simulink model "step05_STM32_ControllerPrep"  (R2024b)
settings: Solver=VariableStepAuto  StartTime=0.0  StopTime=1.5  RelTol=1e-3
libraries: spsSeriesRLCBranchLib x6, spsCurrentMeasurementLib x4, spsUniversalBridgeLib x2, spsVoltageMeasurementLib x2, spsACVoltageSourceLib x1, spsRMSLib x1, slpidlib x1, spspowerguiLib x1
settings Model: Creator=asus  LastModifiedBy=asus

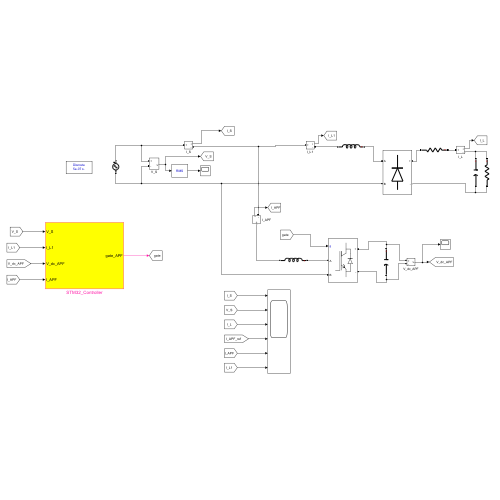
[thumbnail: Simulink's stored preview of the top-level diagram]
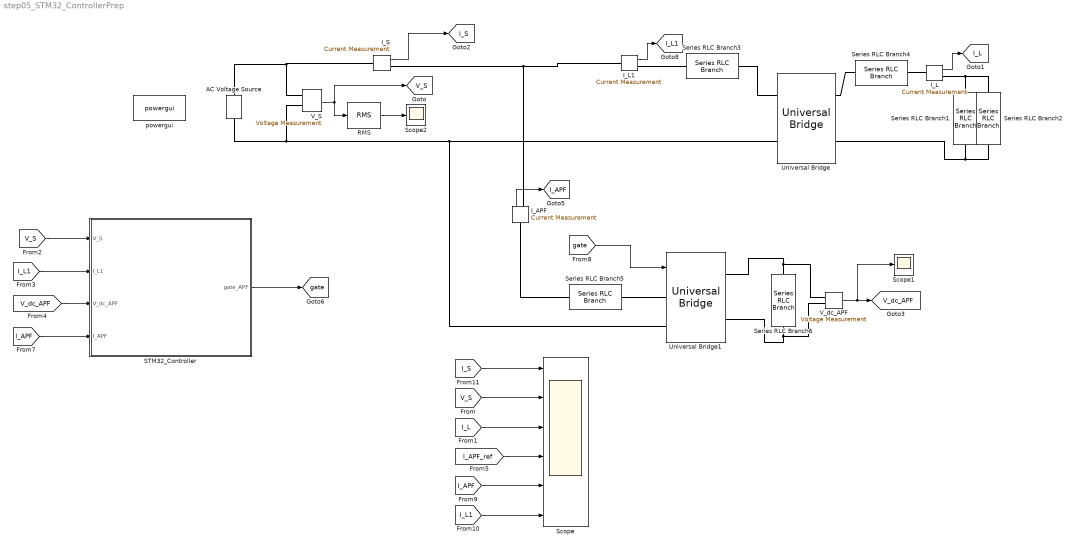
== system step05_STM32_ControllerPrep ==
  AC Voltage Source : spsACVoltageSourceLib/AC Voltage Source  Amplitude=67.88225  Phase=0  Frequency=50  SampleTime=0  Measurements=None  BusType=swing  Pref=10e3  Qref=0  Qmin=-inf  Qmax=+inf
  I_APF : spsCurrentMeasurementLib/Current Measurement  PhasorSimulation=off  OutputType=Complex  PSBequivalent=0
  I_L : spsCurrentMeasurementLib/Current Measurement  PhasorSimulation=off  OutputType=Complex  PSBequivalent=0
  I_L1 : spsCurrentMeasurementLib/Current Measurement  PhasorSimulation=off  OutputType=Complex  PSBequivalent=0
  I_S : spsCurrentMeasurementLib/Current Measurement  PhasorSimulation=off  OutputType=Complex  PSBequivalent=0
  RMS : spsRMSLib/RMS  TrueRMS=on  Freq=50  RMSInit=120  Ts=0
  STM32_Controller : Subsystem
  Scope : Scope  NumInputPorts=6
  Scope1 : Scope
  Scope2 : Scope
  Series RLC Branch1 : spsSeriesRLCBranchLib/Series RLC Branch  LConnTagsString=__new0  RConnTagsString=__new0  BranchType=C  Resistance=30  Inductance=220e-5  SetiL0=off  InitialCurrent=0  Capacitance=100e-5  Setx0=off  InitialVoltage=0  Measurements=None
  Series RLC Branch2 : spsSeriesRLCBranchLib/Series RLC Branch  LConnTagsString=__new0  RConnTagsString=__new0  BranchType=R  Resistance=30  Inductance=0.8  SetiL0=off  InitialCurrent=0  Capacitance=1e-6  Setx0=off  InitialVoltage=0  Measurements=None
  Series RLC Branch3 : spsSeriesRLCBranchLib/Series RLC Branch  LConnTagsString=__new0  RConnTagsString=__new0  BranchType=L  Resistance=0.5  Inductance=2e-2  SetiL0=off  InitialCurrent=0  Capacitance=1e-6  Setx0=off  InitialVoltage=0  Measurements=None
  Series RLC Branch4 : spsSeriesRLCBranchLib/Series RLC Branch  LConnTagsString=__new0  RConnTagsString=__new0  BranchType=R  Resistance=2  Inductance=0.8  SetiL0=off  InitialCurrent=0  Capacitance=1e-6  Setx0=off  InitialVoltage=0  Measurements=None
  Series RLC Branch5 : spsSeriesRLCBranchLib/Series RLC Branch  LConnTagsString=__new0  RConnTagsString=__new0  BranchType=L  Resistance=0.5  Inductance=5e-3  SetiL0=off  InitialCurrent=0  Capacitance=1e-6  Setx0=off  InitialVoltage=0  Measurements=None
  Series RLC Branch6 : spsSeriesRLCBranchLib/Series RLC Branch  LConnTagsString=__new0  RConnTagsString=__new0  BranchType=C  Resistance=30  Inductance=220e-5  SetiL0=off  InitialCurrent=0  Capacitance=5e-3  Setx0=on  InitialVoltage=0  Measurements=None
  Universal Bridge : spsUniversalBridgeLib/Universal Bridge  Arms=2  SnubberResistance=1e5  SnubberCapacitance=1e-6  Device=Diodes  Ron=1e-3  Lon=0  ForwardVoltages="[  0  0  ]"  ForwardVoltage=0  GTOparameters=[ 10e-6 , 20e-6 ]  IGBTparameters=[ 1e-6 , 2e-6 ]  Measurements=None  Measurements_2=None  converterType=Rectifier
  Universal Bridge1 : spsUniversalBridgeLib/Universal Bridge  Arms=2  SnubberResistance=1e5  SnubberCapacitance=1e-6  Device=IGBT / Diodes  Ron=1e-3  Lon=0  ForwardVoltages="[  0  0  ]"  ForwardVoltage=0  GTOparameters=[ 10e-6 , 20e-6 ]  IGBTparameters=[ 1e-6 , 2e-6 ]  Measurements=None  Measurements_2=None  converterType=Rectifier
  V_S : spsVoltageMeasurementLib/Voltage Measurement  PhasorSimulation=off  OutputType=Complex  PSBequivalent=0
  V_dc_APF : spsVoltageMeasurementLib/Voltage Measurement  PhasorSimulation=off  OutputType=Complex  PSBequivalent=0
  powergui : spspowerguiLib/powergui  Priority=1  SimulationMode=Discrete  SampleTime=5e-7  frequency=60  Iterations=50  frequencyindice=50  Pbase=100e6  ErrMax=1e-4  UnitsV=kV  UnitsW=MW  buscounter=0  FunctionMessages=off  echomessages=off  EnableUseOfTLC=off  CurrentSourceSwitches=off  DisableSnubberDevices=off  DisableRonSwitches=off  DisableVfSwitches=off  DisplayEquations=off  AutomaticDiscreteSolvers=off  SolverType=Tustin/Backward Euler (TBE)  Interpol=off  ExternalGateDelay=off  methode=off  Ts=100  x0status=blocks  SPID=on  SwTol=0  HookPort=off  NonlinearTolerance=1e-4  nMaxIteration=100  ContinueOnMaxIteration=off  RestoreLinks=warning  ResistiveCurrentMeasurement=off  Frange=[0:2:500]  Ylog=off  Xlog=on  ShowGrid=off  save=off  variable=ZData  structure=0  ZoomFFT=off  StartTime=0.0  cycles=1  DisplayStyle=1  fundamental=60  FreqAxis=off  MaxFrequency=1000  frequencyindicesteady=1  RmsSteady=1  display=off
  tag scope: I_APF=global, I_L1=global, I_L=global, I_S=global, V_S=global, V_dc_APF=global, gate=global
  wires:
  I_S/1 -> [I_S]
  V_dc_APF/1 -> Scope1/1, [V_dc_APF]
  RMS/1 -> Scope2/1
  [I_L1] -> Scope/6
  [I_S] -> Scope/1
  I_L/1 -> [I_L]
  V_S/1 -> RMS/1, [V_S]
  I_L1/1 -> [I_L1]
  [gate] -> Universal Bridge1/1
  I_APF/1 -> [I_APF]
  [V_S] -> Scope/2
  [I_L] -> Scope/3
  [I_APF_ref] -> Scope/4
  [I_APF] -> Scope/5
  [V_S] -> STM32_Controller/1(V_S)
  [I_L1] -> STM32_Controller/2(I_L1)
  [V_dc_APF] -> STM32_Controller/3(V_dc_APF)
  [I_APF] -> STM32_Controller/4(I_APF)
  STM32_Controller/1(gate_APF) -> [gate]
  connections:
  V_S/LConn2 -- Universal Bridge/LConn2 -- Universal Bridge1/LConn2 -- AC Voltage Source/LConn1
  Universal Bridge1/RConn1 -- Series RLC Branch6/LConn1 -- V_dc_APF/LConn1
  Series RLC Branch2/RConn1 -- Universal Bridge/RConn2 -- Series RLC Branch1/RConn1
  I_S/LConn1 -- V_S/LConn1 -- AC Voltage Source/RConn1
  Universal Bridge1/RConn2 -- Series RLC Branch6/RConn1 -- V_dc_APF/LConn2
  I_S/RConn1 -- I_APF/RConn1 -- I_L1/LConn1
  I_L/RConn1 -- Series RLC Branch2/LConn1 -- Series RLC Branch1/LConn1
  I_L/LConn1 -- Series RLC Branch4/LConn1
  Series RLC Branch5/LConn1 -- Universal Bridge1/LConn1
  Universal Bridge/LConn1 -- Series RLC Branch3/LConn1
  I_L1/RConn1 -- Series RLC Branch3/RConn1
  Series RLC Branch5/RConn1 -- I_APF/LConn1
  Series RLC Branch4/RConn1 -- Universal Bridge/RConn1

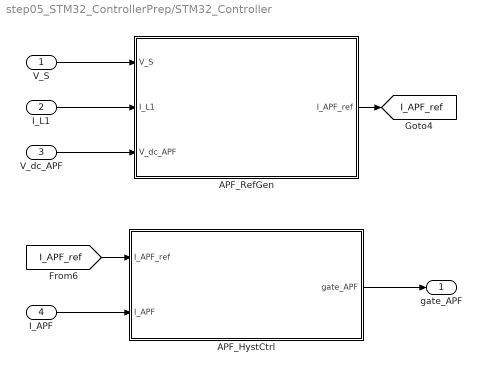
== system step05_STM32_ControllerPrep/STM32_Controller ==
  V_S : Inport
  I_L1 : Inport  Port=2
  V_dc_APF : Inport  Port=3
  I_APF : Inport  Port=4
  APF_HystCtrl : Subsystem
  APF_RefGen : Subsystem
  gate_APF : Outport
  tag scope: I_APF_ref=global
  wires:
  [I_APF_ref] -> APF_HystCtrl/1(I_APF_ref)
  APF_RefGen/1(I_APF_ref) -> [I_APF_ref]
  I_L1/1 -> APF_RefGen/2(I_L1)
  I_APF/1 -> APF_HystCtrl/2(I_APF)
  APF_HystCtrl/1(gate_APF) -> gate_APF/1
  V_S/1 -> APF_RefGen/1(V_S)
  V_dc_APF/1 -> APF_RefGen/3(V_dc_APF)

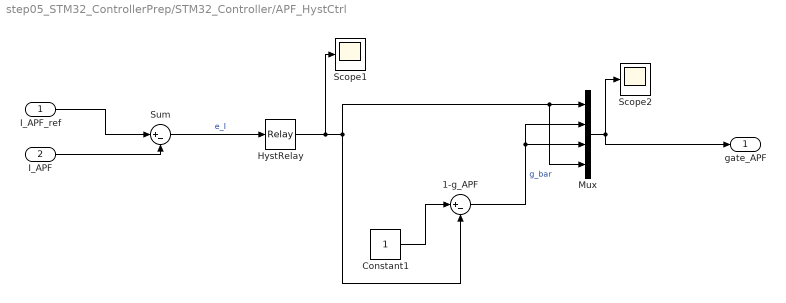
== system step05_STM32_ControllerPrep/STM32_Controller/APF_HystCtrl ==
  I_APF_ref : Inport
  I_APF : Inport  Port=2
  1-g_APF : Sum  Inputs=|+-
  Constant1 : Constant
  HystRelay : Relay  OnSwitchValue=0.1  OffSwitchValue=-0.1
  Mux : Mux
  Scope1 : Scope
  Scope2 : Scope
  Sum : Sum  Inputs=|+-
  gate_APF : Outport
  wires:
  I_APF_ref/1 -> Sum/1
  I_APF/1 -> Sum/2
  Sum/1 -> HystRelay/1  "e_I"
  Constant1/1 -> 1-g_APF/1
  HystRelay/1 -> Scope1/1, Mux/4, Mux/1, 1-g_APF/2
  1-g_APF/1 -> Mux/3, Mux/2  "g_bar"
  Mux/1 -> gate_APF/1, Scope2/1

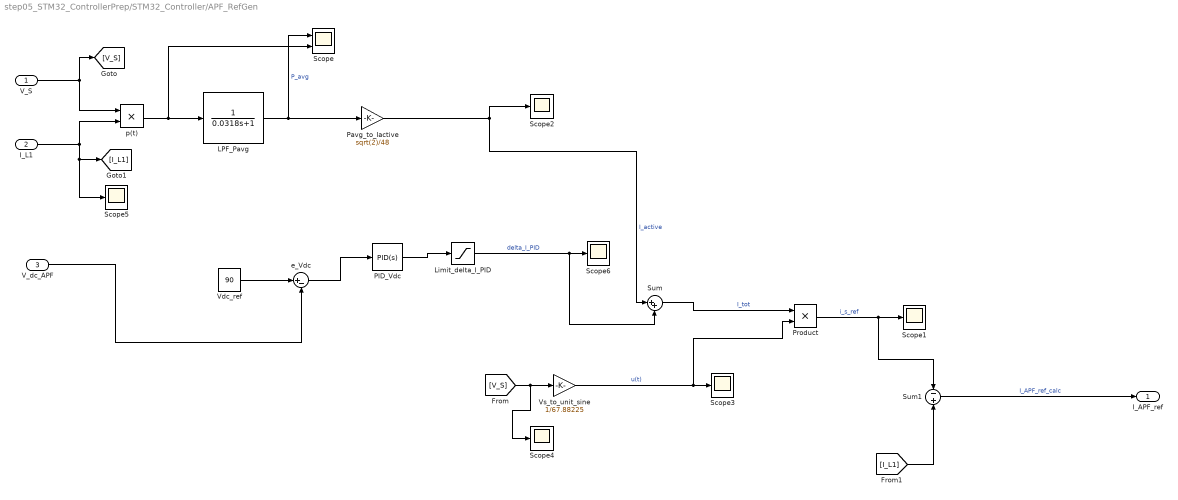
== system step05_STM32_ControllerPrep/STM32_Controller/APF_RefGen ==
  V_S : Inport
  I_L1 : Inport  Port=2
  V_dc_APF : Inport  Port=3
  LPF_Pavg : TransferFcn  Denominator=[0.0318 1]
  Limit_delta_I_PID : Saturate  UpperLimit=1.5  LowerLimit=-1.5
  PID_Vdc : slpidlib/PID Controller  Controller=PID  Form=Parallel  TimeDomain=Continuous-time  UseExternalTs=off  SampleTime=-1  IntegratorMethod=Forward Euler  FilterMethod=Forward Euler  ControllerParametersSource=internal  P=0.5  I=50  UseKiTs=off  D=0  UseExternalDerivativeSource=off  N=100  UseFilter=on  TunerSelectOption=Transfer Function Based (PID Tuner App)  InitialConditionSource=internal  InitialConditionForIntegrator=0  InitialConditionForFilter=0  DifferentiatorICPrevScaledInput=0  ExternalReset=none  TrackingMode=off  Kt=1  LimitOutput=off  SatLimitsSource=internal  UpperSaturationLimit=inf  LowerSaturationLimit=-inf  LinearizeAsGain=on  AntiWindupMode=none  Kb=1  LimitIntegrator=off  UpperIntegratorSaturationLimit=inf  LowerIntegratorSaturationLimit=-inf  POutMin=[]  POutMax=[]  IOutMin=[]  IOutMax=[]  DOutMin=[]  DOutMax=[]  NOutMin=[]  NOutMax=[]  SumOutMin=[]  SumOutMax=[]  SaturationOutMin=[]  SaturationOutMax=[]  PParamMin=[]  PParamMax=[]  IParamMin=[]  IParamMax=[]  DParamMin=[]  DParamMax=[]  NParamMin=[]  NParamMax=[]  KbParamMin=[]  KbParamMax=[]  KtParamMin=[]  KtParamMax=[]  KbOutMin=[]  KbOutMax=[]  KtOutMin=[]  KtOutMax=[]  IntegratorOutMin=[]  IntegratorOutMax=[]  FilterOutMin=[]  FilterOutMax=[]  SumI1OutMin=[]  SumI1OutMax=[]  SumI2OutMin=[]  SumI2OutMax=[]  SumI3OutMin=[]  SumI3OutMax=[]  SumI4OutMin=[]  SumI4OutMax=[]  SumDOutMin=[]  SumDOutMax=[]  DifferentiatorOutMin=[]  DifferentiatorOutMax=[]  FilterDiffOutCoefMin=[]  FilterDiffOutCoefMax=[]  ReciprocalOutMin=[]  ReciprocalOutMax=[]  SumDenOutMin=[]  SumDenOutMax=[]  SumNumOutMin=[]  SumNumOutMax=[]  DivideOutMin=[]  DivideOutMax=[]  UdiffTsProdOutMin=[]  UdiffTsProdOutMax=[]  NTsProdOutMin=[]  NTsProdOutMax=[]  UintegralTsProdOutMin=[]  UintegralTsProdOutMax=[]  UngainTsProdOutMin=[]  UngainTsProdOutMax=[]  ClampingZeroOutDataTypeStr=Inherit: Inherit via back propagation  ClampingZeroOutMin=[]  ClampingZeroOutMax=[]  FilterDenConstantOutDataTypeStr=Inherit: Inherit via back propagation  FilterDenConstantOutMin=[]  FilterDenConstantOutMax=[]  PCopyOutDataTypeStr=Inherit: Inherit via back propagation  PCopyOutMin=[]  PCopyOutMax=[]  NCopyOutDataTypeStr=Inherit: Inherit via back propagation  NCopyOutMin=[]  NCopyOutMax=[]  IntegratorContinuousStateAttributes=''  IntegratorStateMustResolveToSignalObject=off  IntegratorRTWStateStorageClass=Auto  FilterContinuousStateAttributes=''  FilterStateMustResolveToSignalObject=off  FilterRTWStateStorageClass=Auto  ParallelPVariant=InternalParameters  IdealPVariant=Disabled  IVariant=InternalParameters  DVariant=InternalParameters  IntegratorVariant=Continuous  SatVariant=Disabled  AWVariant=Passthrough  PCopyVariant=Disabled  TRVariant=Disabled  FdbkBlocksVariant=Forward  IdealPFdbkVariant=Disabled  SatFdbkVariant=Disabled  DerivativeFilterVariant=ContFilter  NVariant=InternalParameters  NCopyVariant=Disabled  FilterICVariant=InternalICsFilter  IntegratorICVariant=InternalICs  ExternalResetVariant=Disabled  TRSumVariant=Passthrough  SumFdbkVariant=Disabled  SumVariant=Sum_PID  TsampFilterVariant=InternalTs  TsampNgainVariant=Passthrough  TsampIntegralVariant=Disabled_SignalSpec  ExternalSaturationOutDataTypeStr=Inherit: Same as second input  DerivativeSourceVariant=ErrorSignal  PreIntVariant=InternalPreInt
  Pavg_to_Iactive : Gain  Gain=sqrt(2)/48
  Product : Product
  Scope : Scope  NumInputPorts=2
  Scope{1..6} (6 alike) : Scope
  Sum : Sum  Inputs=|++
  Sum1 : Sum  Inputs=-+
  Vdc_ref : Constant  Value=90
  Vs_to_unit_sine : Gain  Gain=1/67.88225
  e_Vdc : Sum  Inputs=|+-
  p(t) : Product
  I_APF_ref : Outport
  wires:
  p(t)/1 -> Scope/2, LPF_Pavg/1
  LPF_Pavg/1 -> Pavg_to_Iactive/1, Scope/1  "P_avg"
  Pavg_to_Iactive/1 -> Sum/1, Scope2/1  "I_active"
  Vdc_ref/1 -> e_Vdc/1
  V_dc_APF/1 -> e_Vdc/2
  e_Vdc/1 -> PID_Vdc/1
  PID_Vdc/1 -> Limit_delta_I_PID/1
  Limit_delta_I_PID/1 -> Sum/2, Scope6/1  "delta_I_PID"
  Sum/1 -> Product/1  "I_tot"
  [V_S] -> Scope4/1, Vs_to_unit_sine/1
  V_S/1 -> p(t)/1, [V_S]
  Vs_to_unit_sine/1 -> Scope3/1, Product/2  "u(t)"
  Product/1 -> Sum1/1, Scope1/1  "i_s_ref"
  [I_L1] -> Sum1/2
  Sum1/1 -> I_APF_ref/1  "I_APF_ref_calc"
  I_L1/1 -> Scope5/1, [I_L1], p(t)/2
